simulink model "verify_HeatTransfer2Ground_ISO13370_mdl"  (R2016b)
settings: Solver=ode45  StartTime=0  StopTime=365*24*3600  MaxStep=24*3600  RelTol=1e-3  EnableMultiTasking=on
libraries: carnot x1
settings Model: Creator=drhf  LastModifiedBy=srrt
settings DataIOCC: SaveFormat=Array  SignalLoggingSaveFormat=ModelDataLogs
settings OptimizationCC: ExpressionDepthLimit=2147483647  LifeSpan=inf
settings DebuggingCC: UnderspecifiedInitializationDetection=Classic  MergeDetectMultiDrivingBlocksExec=none  SolverPrmCheckMsg=warning  FcnCallInpInsideContextMsg=warning  StateNameClashWarn=warning  SFUnexpectedBacktrackingDiag=warning  SFNoUnconditionalDefaultTransitionDiag=warning  SFExecutionAtInitializationDiag=none
settings HardwareCC: ProdBitPerPointer=32  ProdBitPerSizeT=32  ProdBitPerPtrDiffT=32  ProdLargestAtomicFloat=None  ProdIntDivRoundTo=Undefined  ProdEndianess=Unspecified  ProdWordSize=32  ProdHWDeviceType=32-bit Generic
settings ModelReferenceCC: PropagateSignalLabelsOutOfModel=off
settings GRTTargetCC: TargetLangStandard=C89/C90 (ANSI)  GeneratePreprocessorConditionals=Disable all  CombineOutputUpdateFcns=off  GRTInterface=on
settings ConfigComp: CovMetricSettings=dw  CovHtmlReporting=on  CovSaveCumulativeToWorkspaceVar=on  CovSaveSingleToWorkspaceVar=on  CovExternalEMLEnable=off

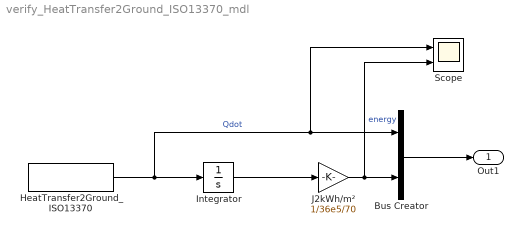
== system verify_HeatTransfer2Ground_ISO13370_mdl ==
  Bus Creator : BusCreator  Inputs=2
  HeatTransfer2Ground_ISO13370 : carnot/Load/Houses/heat_transfer/HeatTransfer2Ground_ISO13370  wallsize=[7 10]  gammat=0  Tmeaninside=23.8  deltathetai=3.8  Tmeanoutside=11  deltathetae=9.3  tshift=319*3600  dwall=0.4  cond_ground=2.0  cp_ground=800  rho_ground=2500  rtot=1./0.183
  Integrator : Integrator
  J2kWh/m² : Gain  Gain=1/36e5/70
  Scope : Scope  NumInputPorts=2
  Out1 : Outport
  wires:
  Integrator/1 -> J2kWh/m²/1
  HeatTransfer2Ground_ISO13370/1 -> Scope/1, Bus Creator/1, Integrator/1  "Qdot"
  J2kWh/m²/1 -> Scope/2, Bus Creator/2  "energy"
  Bus Creator/1 -> Out1/1
